simulink model "controller"  (R2020b)
settings: Solver=ode8  StartTime=0.0  StopTime=inf  FixedStep=0.01  RelTol=1e-3
undefined symbols (not defined in the file or in its folder): Acceleration, Jerk, Speed, SteeringAngle, SteeringAngleVelocity
libraries: robotlib x6, drivingvehiclecontroller x2, simulink_extras x1
settings Model: Creator=hmcl  LastModifiedBy=hmcl
settings OptimizationCC: EnhancedBackFolding=on  PassReuseOutputArgsAs=Individual arguments  ZeroExternalMemoryAtStartup=off  ZeroInternalMemoryAtStartup=off  MaxStackSize=64  OptimizeBlockOrder=speed  DifferentSizesBufferReuse=on  OptimizationCustomize=off  EfficientTunableParamExpr=on
settings DebuggingCC: ParameterTunabilityLossMsg=error
settings HardwareCC: ProdBitPerPointer=32  ProdBitPerSizeT=32  ProdBitPerPtrDiffT=32  ProdLargestAtomicFloat=None  ProdIntDivRoundTo=Undefined  ProdEndianess=Unspecified  ProdWordSize=32  ProdHWDeviceType=Generic->Unspecified (assume 32-bit Generic)
settings SFSimCC: MATLABDynamicMemAlloc=off  SimTargetLang=C++
settings RTWCC: Description=Embedded Coder  SystemTargetFile=ert.tlc  HardwareBoard=Robot Operating System (ROS)  TLCOptions="-aInlineSetEventsForThisBaseRateFcn=TLC_FALSE -aSuppressMultiTaskScheduler=TLC_FALSE  -aRateBasedStepFcn=0"  GenCodeOnly=on  TemplateMakefile=ert_default_tmf  RTWVerbose=off  Toolchain=Catkin  TargetLang=C++
settings CodeAppCC: ForceParamTrailComments=on  IgnoreCustomStorageClasses=off  OperatorAnnotations=on  SimulinkDataObjDesc=on  SFDataObjDesc=on  InsertBlockDesc=on

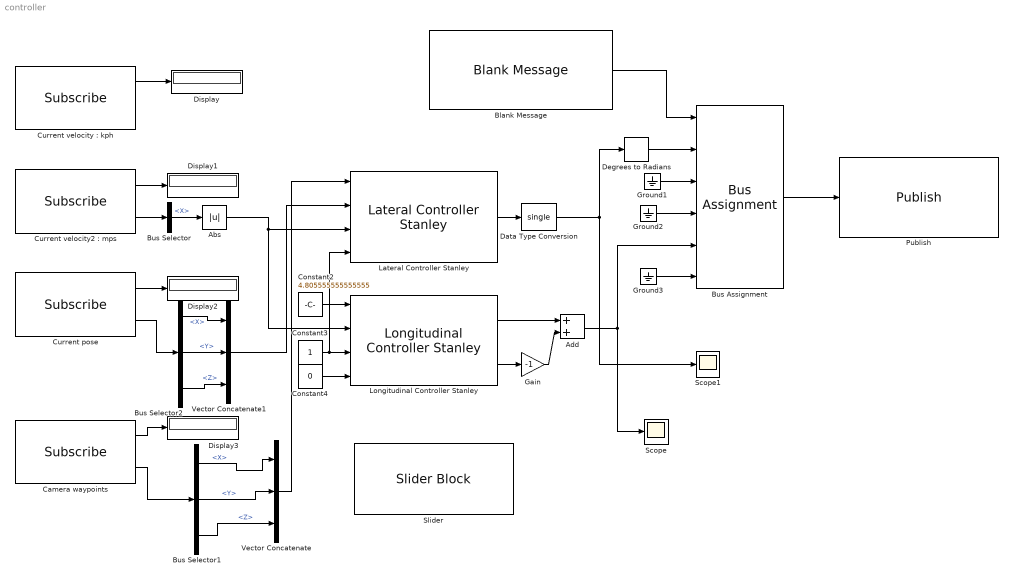
== system controller ==
  Abs : Abs
  Add : Sum  OutDataTypeStr=single
  Blank Message : robotlib/Blank Message  messageClass=Message  entityType=ackermann_msgs/AckermannDrive  messageType=ackermann_msgs/AckermannDrive  SampleTime=-1  legacyBusStruct=off
  Bus Assignment : BusAssignment  AssignedSignals=SteeringAngle,SteeringAngleVelocity,Speed,Acceleration,Jerk
  Bus Selector : BusSelector  OutputSignals=Twist.Linear.X
  Bus Selector1 : BusSelector  OutputSignals=X,Y,Z
  Bus Selector2 : BusSelector  OutputSignals=X,Y,Z
  Camera waypoints : robotlib/Subscribe  topicSource=Select from ROS network  topic=/nearest_waypoint  messageType=geometry_msgs/Vector3  SampleTime=-1  legacyBusStruct=off  messageQueueLength=1
  Constant2 : Constant  Value=4.805555555555555
  Constant3 : Constant
  Constant4 : Constant  Value=0
  Current pose : robotlib/Subscribe  topicSource=Select from ROS network  topic=/gnss_pose_relay  messageType=geometry_msgs/Vector3  SampleTime=-1  legacyBusStruct=off  messageQueueLength=1
  "Current velocity : kph" : robotlib/Subscribe  topicSource=Select from ROS network  topic=/estimated_vel_kmph  messageType=std_msgs/Float32  SampleTime=-1  legacyBusStruct=off  messageQueueLength=1
  "Current velocity2 : mps" : robotlib/Subscribe  topicSource=Select from ROS network  topic=/current_velocity  messageType=geometry_msgs/TwistStamped  SampleTime=-1  legacyBusStruct=off  messageQueueLength=1
  Data Type Conversion : DataTypeConversion  OutDataTypeStr=single
  Degrees to Radians : simulink_extras/Transformations/Degrees to Radians
  Display{,1..3} (4 alike) : Display
  Gain : Gain  Gain=-1
  Ground1 : Ground
  Ground2 : Ground
  Ground3 : Ground
  Lateral Controller Stanley : drivingvehiclecontroller/Lateral Controller Stanley  ModelType=Kinematic bicycle model  PositionGainF=2.0  PositionGainR=2.5  YawRateGain=0.2  DelayGain=0.2  VehicleMass=1575  Lf=1.2  Lr=1.6  TireStiffness=19000  Wheelbase=2.8  MaxSteeringAngle=35
      settings: SourceProductBaseCode=DR
  Longitudinal Controller Stanley : drivingvehiclecontroller/Longitudinal Controller Stanley  Kp=0.1  Ki=0.1  SampleTime=0.05  MaxAcceleration=3  MaxDeceleration=6
      settings: SourceProductBaseCode=DR
  Publish : robotlib/Publish  topicSource=Select from ROS network  topic=/carla/ego_vehicle/ackermann_cmd  messageType=ackermann_msgs/AckermannDrive  legacyBusStruct=off  messageQueueLength=1
  Scope : Scope
  Scope1 : Scope
  Slider : SliderBlock  ScaleMax=40
  Vector Concatenate : Concatenate  NumInputs=3
  Vector Concatenate1 : Concatenate  NumInputs=3
  wires:
  Blank Message/1 -> Bus Assignment/1
  Bus Assignment/1 -> Publish/1
  Lateral Controller Stanley/1 -> Data Type Conversion/1
  Ground1/1 -> Bus Assignment/3
  Add/1 -> Scope/1, Bus Assignment/5
  Ground2/1 -> Bus Assignment/4
  Ground3/1 -> Bus Assignment/6
  "Current velocity : kph"/1 -> Display/1
  "Current velocity2 : mps"/1 -> Display1/1
  Current pose/1 -> Display2/1
  Camera waypoints/1 -> Display3/1
  Constant2/1 -> Longitudinal Controller Stanley/1
  "Current velocity2 : mps"/2 -> Bus Selector/1
  Bus Selector/1 -> Abs/1  "<X>"
  Constant3/1 -> Longitudinal Controller Stanley/3, Lateral Controller Stanley/4
  Constant4/1 -> Longitudinal Controller Stanley/4
  Longitudinal Controller Stanley/1 -> Add/1
  Longitudinal Controller Stanley/2 -> Gain/1
  Gain/1 -> Add/2
  Camera waypoints/2 -> Bus Selector1/1
  Bus Selector1/2 -> Vector Concatenate/2  "<Y>"
  Bus Selector1/1 -> Vector Concatenate/1  "<X>"
  Bus Selector1/3 -> Vector Concatenate/3  "<Z>"
  Vector Concatenate/1 -> Lateral Controller Stanley/1
  Current pose/2 -> Bus Selector2/1
  Bus Selector2/1 -> Vector Concatenate1/1  "<X>"
  Bus Selector2/2 -> Vector Concatenate1/2  "<Y>"
  Bus Selector2/3 -> Vector Concatenate1/3  "<Z>"
  Vector Concatenate1/1 -> Lateral Controller Stanley/2
  Data Type Conversion/1 -> Scope1/1, Degrees to Radians/1
  Abs/1 -> Longitudinal Controller Stanley/2, Lateral Controller Stanley/3
  Degrees to Radians/1 -> Bus Assignment/2
